simulink model "check_for_update"  (R2023b)
settings: Solver=FixedStepAuto  StartTime=0.0  StopTime=t(end)  FixedStep=1  RelTol=1e-3
libraries: nav_lib x1
settings Model: Creator=brent  LastModifiedBy=brent

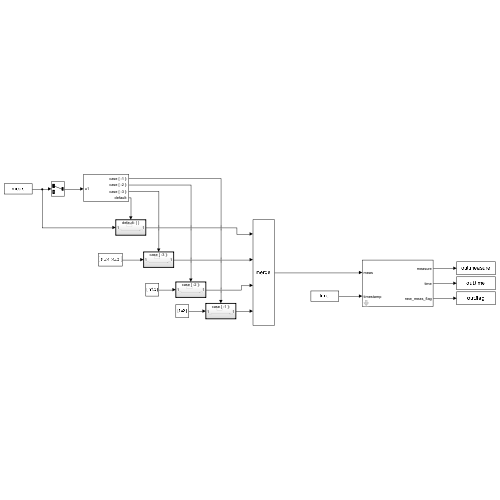
[thumbnail: Simulink's stored preview of the top-level diagram]
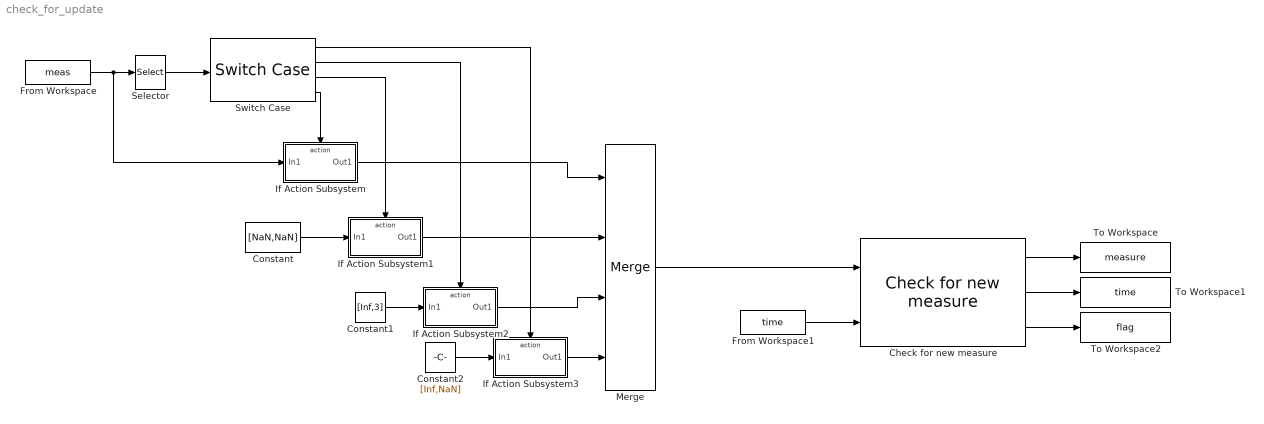
== system check_for_update ==
  Check for new measure : nav_lib/Check for new measure
      settings: SourceProductName=Navigation library
  Constant : Constant  Value=[NaN,NaN]
  Constant1 : Constant  Value=[Inf,3]
  Constant2 : Constant  Value=[Inf,NaN]
  From Workspace : FromWorkspace  VariableName=meas  OutputAfterFinalValue=Holding final value
  From Workspace1 : FromWorkspace  VariableName=time
  If Action Subsystem : Subsystem  TreatAsAtomicUnit=on
  If Action Subsystem1 : Subsystem  TreatAsAtomicUnit=on
  If Action Subsystem2 : Subsystem  TreatAsAtomicUnit=on
  If Action Subsystem3 : Subsystem  TreatAsAtomicUnit=on
  Merge : Merge  Inputs=4
  Selector : Selector  InputPortWidth=2  IndexOptions=Index vector (dialog)  Indices=1  OutputSizes=1
  Switch Case : SwitchCase  CaseConditions={-1,-2,-3}
  To Workspace : ToWorkspace  VariableName=measure  SampleTime=-1
      settings: Save2DSignal=2-D array (concatenate along first dimension)
  To Workspace1 : ToWorkspace  VariableName=time  SampleTime=-1
      settings: Save2DSignal=2-D array (concatenate along first dimension)
  To Workspace2 : ToWorkspace  VariableName=flag  SampleTime=-1
      settings: Save2DSignal=2-D array (concatenate along first dimension)
  wires:
  If Action Subsystem2/1(Out1) -> Merge/3
  If Action Subsystem3/1(Out1) -> Merge/4
  Switch Case/1 -> If Action Subsystem3/Action
  Switch Case/4 -> If Action Subsystem/Action
  Check for new measure/1 -> To Workspace/1
  From Workspace/1 -> If Action Subsystem/1(In1), Selector/1
  Check for new measure/2 -> To Workspace1/1
  Selector/1 -> Switch Case/1
  Check for new measure/3 -> To Workspace2/1
  From Workspace1/1 -> Check for new measure/2
  Merge/1 -> Check for new measure/1
  Switch Case/3 -> If Action Subsystem1/Action
  Constant1/1 -> If Action Subsystem2/1(In1)
  Constant/1 -> If Action Subsystem1/1(In1)
  Switch Case/2 -> If Action Subsystem2/Action
  If Action Subsystem1/1(Out1) -> Merge/2
  Constant2/1 -> If Action Subsystem3/1(In1)
  If Action Subsystem/1(Out1) -> Merge/1

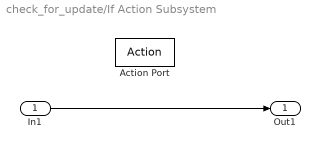
== system check_for_update/If Action Subsystem ==
  In1 : Inport
  Action Port : ActionPort  ActionPortLabel=default:
  Out1 : Outport
  wires:
  In1/1 -> Out1/1

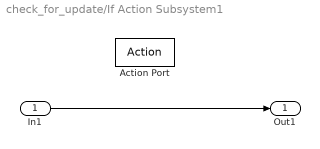
== system check_for_update/If Action Subsystem1 ==
  In1 : Inport
  Action Port : ActionPort  ActionPortLabel=case [ -3 ]:
  Out1 : Outport
  wires:
  In1/1 -> Out1/1

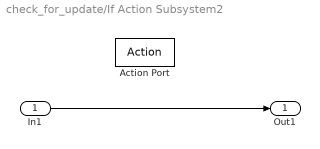
== system check_for_update/If Action Subsystem2 ==
  In1 : Inport
  Action Port : ActionPort  ActionPortLabel=case [ -2 ]:
  Out1 : Outport
  wires:
  In1/1 -> Out1/1

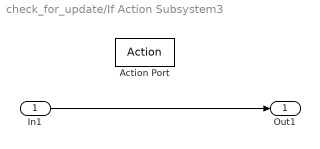
== system check_for_update/If Action Subsystem3 ==
  In1 : Inport
  Action Port : ActionPort  ActionPortLabel=case [ -1 ]:
  Out1 : Outport
  wires:
  In1/1 -> Out1/1
